simulink model "model3"  (R2022b)
settings: Solver=VariableStepAuto  StartTime=0.0  StopTime=10.0  RelTol=1e-3
values from neighbouring files (symbols this model uses):
  a21 = 1/2/m * x30^2 * FemP1/FemP2^2 * exp(-x10/FemP2)    [init.m]    (also in proj.m)
  a23 = -1/m * x30 * FemP1/FemP2 * exp(-x10/FemP2)    [init.m]    (also in proj.m)
  a31 = 1/f1 * exp(x10/f2) * (ki*u10 + ci - x30)    [init.m]    (also in proj.m)
  a33 = -f2/f1 * exp(x10/f2)    [init.m]    (also in proj.m)
  b31 = ki * f2/f1 * exp(x10/f2)    [init.m]    (also in proj.m)
  g = 9.81    [init.m]    (also in proj.m)
settings Model: Creator=pzach  LastModifiedBy=pzach

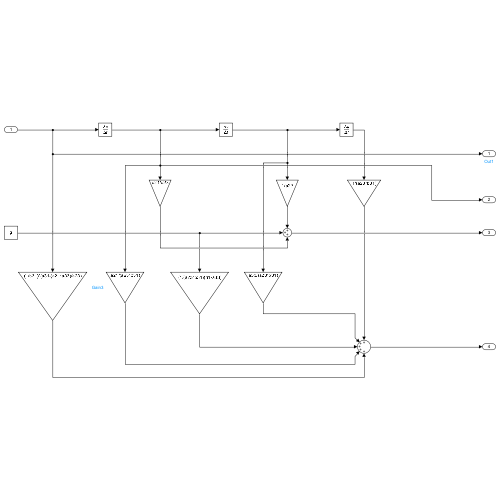
[thumbnail: Simulink's stored preview of the top-level diagram]
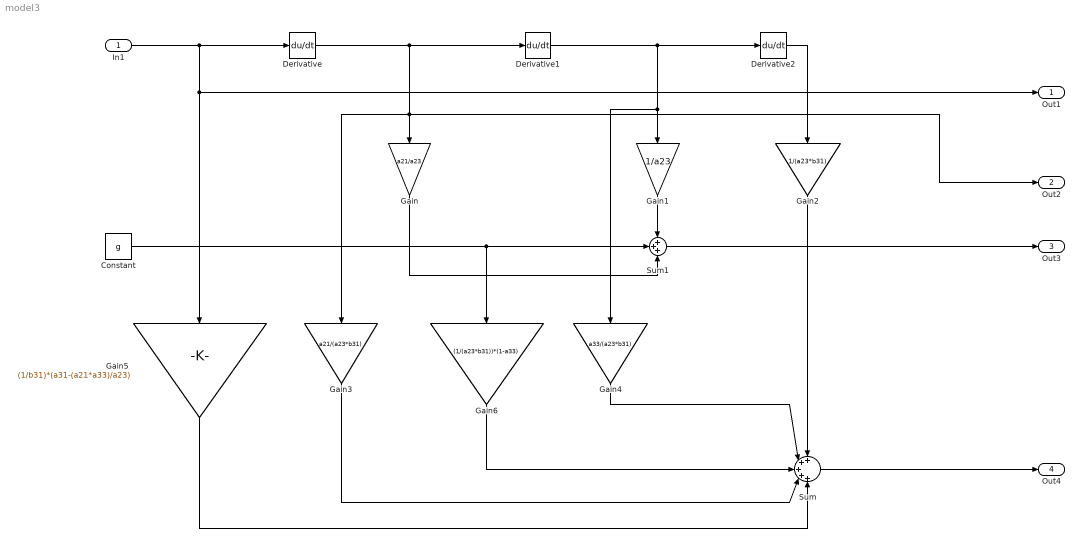
== system model3 ==
  In1 : Inport
  Constant : Constant  Value=g
  Derivative : Derivative
  Derivative1 : Derivative
  Derivative2 : Derivative
  Gain : Gain  Gain=a21/a23
  Gain1 : Gain  Gain=1/a23
  Gain2 : Gain  Gain=1/(a23*b31)
  Gain3 : Gain  Gain=a21/(a23*b31)
  Gain4 : Gain  Gain=a33/(a23*b31)
  Gain5 : Gain  Gain=(1/b31)*(a31-(a21*a33)/a23)
  Gain6 : Gain  Gain=(1/(a23*b31))*(1-a33)
  Sum : Sum  Inputs=+++++
  Sum1 : Sum  Inputs=+++
  Out1 : Outport
  Out2 : Outport  Port=2
  Out3 : Outport  Port=3
  Out4 : Outport  Port=4
  wires:
  Derivative/1 -> Gain3/1, Out2/1, Gain/1, Derivative1/1
  Derivative1/1 -> Gain4/1, Gain1/1, Derivative2/1
  In1/1 -> Out1/1, Gain5/1, Derivative/1
  Gain/1 -> Sum1/3
  Constant/1 -> Gain6/1, Sum1/2
  Gain1/1 -> Sum1/1
  Gain2/1 -> Sum/1
  Derivative2/1 -> Gain2/1
  Sum1/1 -> Out3/1
  Sum/1 -> Out4/1
  Gain4/1 -> Sum/2
  Gain6/1 -> Sum/3
  Gain3/1 -> Sum/4
  Gain5/1 -> Sum/5
